simulink model "Assignment1_2017"  (R2017b)
settings: Solver=FixedStepAuto  StartTime=0.0  StopTime=inf  FixedStep=1E-3  RelTol=1e-3  EnableMultiTasking=on
undefined symbols (not defined in the file): D10, D11, D12, D2, D5, D8, D9, PTA0, PTA2, PTB9, PTC4, PTD0, PTD2, PTD3
libraries: frdmk64flib x8
settings Model: ExtModeTrigDuration=5  Creator=Hassan  LastModifiedBy=Hassan
settings OptimizationCC: EnhancedBackFolding=on  PassReuseOutputArgsAs=Individual arguments  MaxStackSize=64  OptimizeBlockOrder=speed  DifferentSizesBufferReuse=on
settings DebuggingCC: ParameterTunabilityLossMsg=error
settings HardwareCC: ProdBitPerPointer=32  ProdBitPerSizeT=32  ProdBitPerPtrDiffT=32  ProdLargestAtomicInteger=Long  ProdLargestAtomicFloat=Double  ProdWordSize=32  ProdHWDeviceType=ARM Compatible->ARM Cortex  UseEmbeddedCoderFeatures=off
settings SFSimCC: SimUseLocalCustomCode=on  MATLABDynamicMemAlloc=off
settings RTWCC: SystemTargetFile=ert.tlc  HardwareBoard=NXP FRDM-K64F  TemplateMakefile=ert_default_tmf  GenerateReport=on  RTWUseLocalCustomCode=on  Toolchain=GNU Tools for ARM Embedded Processors  IncludeHyperlinkInReport=on  LaunchReport=on  GenerateTraceInfo=on  GenerateTraceReport=on  GenerateTraceReportSl=on  GenerateTraceReportSf=on  GenerateTraceReportEml=on
settings CodeAppCC: ForceParamTrailComments=on  IgnoreCustomStorageClasses=off  OperatorAnnotations=on  SimulinkDataObjDesc=on  SFDataObjDesc=on  InsertBlockDesc=on
settings ERTTargetCC: SupportNonInlinedSFcns=on

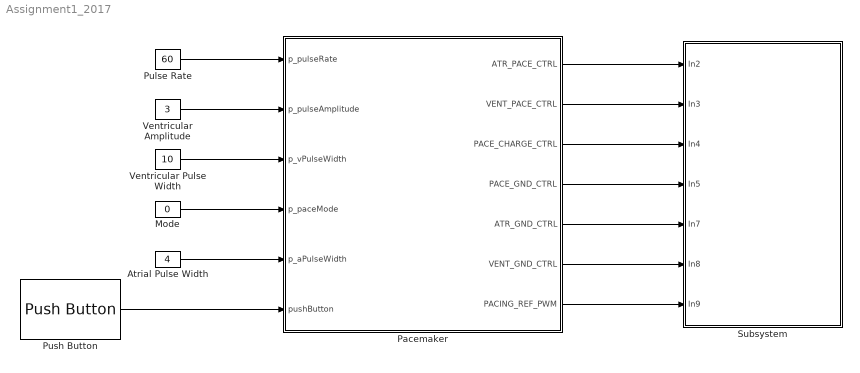
== system Assignment1_2017 ==
  Atrial Pulse Width : Constant  Value=4  OutDataTypeStr=double
  Mode : Constant  Value=0  OutDataTypeStr=uint8
  Pacemaker : Stateflow chart  TreatAsAtomicUnit=on
  Pulse Rate : Constant  Value=60  OutDataTypeStr=double
  Push Button : frdmk64flib/Push Button  Whichswitch=SW3  SampleTime1=-1
      settings: SourceProductName=Simulink Coder Support Package for NXP FRDM-K64F Board
  Subsystem : Subsystem
  Ventricular Amplitude : Constant  Value=3  OutDataTypeStr=double
  Ventricular Pulse Width : Constant  Value=10  OutDataTypeStr=double
  wires:
  Pacemaker/1(ATR_PACE_CTRL) -> Subsystem/1(In2)
  Pacemaker/2(VENT_PACE_CTRL) -> Subsystem/2(In3)
  Pacemaker/3(PACE_CHARGE_CTRL) -> Subsystem/3(In4)
  Pacemaker/4(PACE_GND_CTRL) -> Subsystem/4(In5)
  Pacemaker/5(ATR_GND_CTRL) -> Subsystem/5(In7)
  Pacemaker/6(VENT_GND_CTRL) -> Subsystem/6(In8)
  Ventricular Pulse Width/1 -> Pacemaker/3(p_vPulseWidth)
  Ventricular Amplitude/1 -> Pacemaker/2(p_pulseAmplitude)
  Mode/1 -> Pacemaker/4(p_paceMode)
  Pulse Rate/1 -> Pacemaker/1(p_pulseRate)
  Pacemaker/7(PACING_REF_PWM) -> Subsystem/7(In9)
  Atrial Pulse Width/1 -> Pacemaker/5(p_aPulseWidth)
  Push Button/1 -> Pacemaker/6(pushButton)

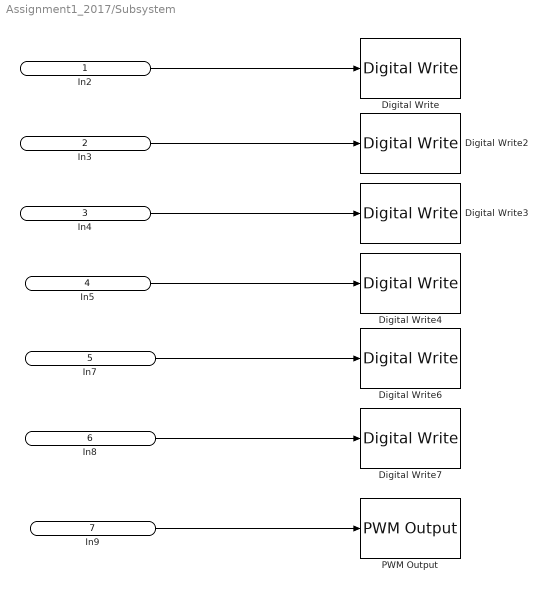
== system Assignment1_2017/Subsystem ==
  In2 : Inport
  In3 : Inport  Port=2
  In4 : Inport  Port=3
  In5 : Inport  Port=4
  In7 : Inport  Port=5
  In8 : Inport  Port=6
  In9 : Inport  Port=7
  Digital Write : frdmk64flib/Digital Write  Whichpin=PTA0 (D8)
      settings: SourceProductName=Simulink Coder Support Package for NXP FRDM-K64F Board
  Digital Write2 : frdmk64flib/Digital Write  Whichpin=PTC4 (D9)
      settings: SourceProductName=Simulink Coder Support Package for NXP FRDM-K64F Board
  Digital Write3 : frdmk64flib/Digital Write  Whichpin=PTB9 (D2)
      settings: SourceProductName=Simulink Coder Support Package for NXP FRDM-K64F Board
  Digital Write4 : frdmk64flib/Digital Write  Whichpin=PTD0 (D10)
      settings: SourceProductName=Simulink Coder Support Package for NXP FRDM-K64F Board
  Digital Write6 : frdmk64flib/Digital Write  Whichpin=PTD2 (D11)
      settings: SourceProductName=Simulink Coder Support Package for NXP FRDM-K64F Board
  Digital Write7 : frdmk64flib/Digital Write  Whichpin=PTD3 (D12)
      settings: SourceProductName=Simulink Coder Support Package for NXP FRDM-K64F Board
  PWM Output : frdmk64flib/PWM Output  Whichpin=PTA2 (D5)  InitialFrequency=1000  InitialDutyCycle=0
      settings: SourceProductName=Simulink Coder Support Package for NXP FRDM-K64F Board
  wires:
  In2/1 -> Digital Write/1
  In3/1 -> Digital Write2/1
  In4/1 -> Digital Write3/1
  In5/1 -> Digital Write4/1
  In7/1 -> Digital Write6/1
  In8/1 -> Digital Write7/1
  In9/1 -> PWM Output/1

== stateflow chart Assignment1_2017/Pacemaker ==
  state ChargeC22DischargeC21
    % Charging C22 and discharging C21
    entry:
    % Charge C22
    VENT_PACE_CTRL=0;
    PACING_REF_PWM=(p_pulseAmplitude/5.0)*100;
    PACE_CHARGE_CTRL=1;
    %Discharge C21
    PACE_GND_CTRL=1;
    VENT_GND_CTRL=1;
  state PaceAtrium
    %PACE ATRIUM
    entry:
    PACE_CHARGE_CTRL=0;
    PACE_GND_CTRL=1;
    ATR_GND_CTRL=0;
    ATR_PACE_CTRL=1;
  state PaceVentricle
    %PACE VENTRICLE
    entry:
    PACE_CHARGE_CTRL=0;
    PACE_GND_CTRL=1;
    VENT_GND_CTRL=0;
    VENT_PACE_CTRL=1;
  state NaturalBeatDetected
    %Going into this state and back
    % to charge state "resets" timer
    % for pacing
  (default) -> ChargeC22DischargeC21
  ChargeC22DischargeC21 -> PaceAtrium [order 3] : [pushButton==0 && p_paceMode==1 && after((60000/p_pulseRate)-p_aPulseWidth, msec)]
  PaceAtrium -> ChargeC22DischargeC21 : [ p_paceMode==1 && after(p_aPulseWidth,msec)]
  ChargeC22DischargeC21 -> PaceVentricle [order 2] : [pushButton==0 && p_paceMode==0 && after((60000/p_pulseRate)-p_vPulseWidth, msec)]
  PaceVentricle -> ChargeC22DischargeC21 : [p_paceMode==0 && after(p_vPulseWidth,msec)]
  ChargeC22DischargeC21 -> NaturalBeatDetected [order 1] : [pushButton==1]
  NaturalBeatDetected -> ChargeC22DischargeC21
  data: p_pulseRate input double; ATR_PACE_CTRL output uint8; VENT_PACE_CTRL output uint8; PACE_CHARGE_CTRL output uint8; PACE_GND_CTRL output uint8; ATR_GND_CTRL output uint8; VENT_GND_CTRL output uint8; p_pulseAmplitude input double; p_vPulseWidth input double; p_paceMode input uint8; p_aPulseWidth input double; PACING_REF_PWM output double; pushButton input boolean
